simulink model "Dong2015IEEECST1"  (R2016b)
settings: Solver=VariableStepAuto  StartTime=0.0001  StopTime=180  FixedStep=0.01  RelTol=1e-6  AbsTol=1e-6
undefined symbols (not defined in the file or in its folder): A, A_xi, B_h, b_h, B_hv, b_hv, B_xi, dfcn_ht, fcn_ht, fcn_xi, theta0, theta1, xi0
settings Model: Creator=xxx  LastModifiedBy=xxx

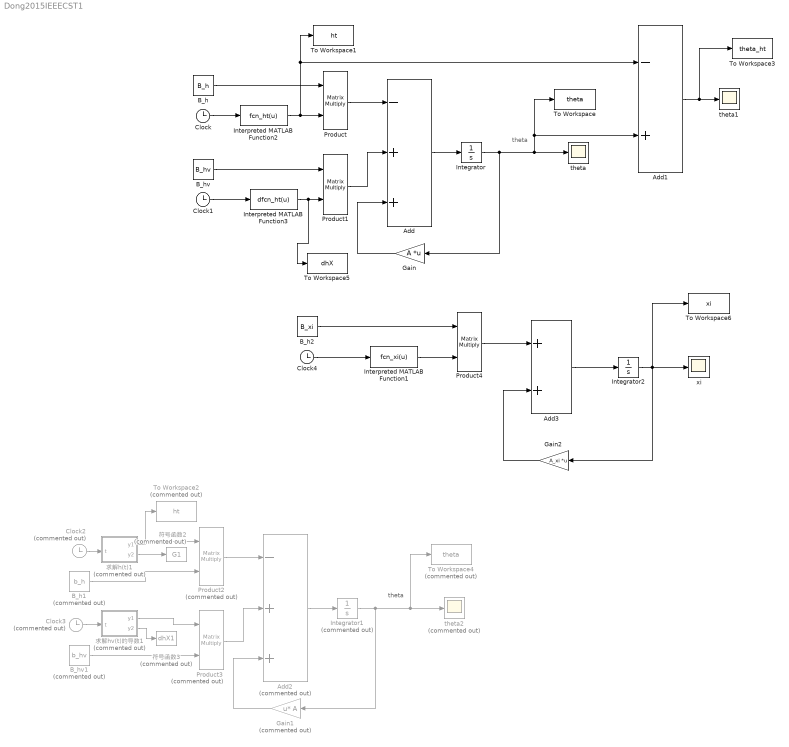
== system Dong2015IEEECST1 ==
  note: theta
  note: theta
  Add : Sum  Inputs=-++
  Add1 : Sum  Inputs=-+
  Add2 : Sum  Commented=on  Inputs=-++
  Add3 : Sum
  B_h : Constant  Value=B_h
  B_h1 : Constant  Commented=on  Value=b_h
  B_h2 : Constant  Value=B_xi
  B_hv : Constant  Value=B_hv
  B_hv1 : Constant  Commented=on  Value=b_hv
  Clock : Clock
  Clock1 : Clock
  Clock2 : Clock  Commented=on
  Clock3 : Clock  Commented=on
  Clock4 : Clock
  Gain : Gain  Gain=A  Multiplication=Matrix(K*u)
  Gain1 : Gain  Commented=on  Gain=A  Multiplication=Matrix(u*K)
  Gain2 : Gain  Gain=A_xi  Multiplication=Matrix(K*u)
  Integrator : Integrator  InitialCondition=theta0
  Integrator1 : Integrator  Commented=on  InitialCondition=theta1
  Integrator2 : Integrator  InitialCondition=xi0
  Interpreted MATLAB Function1 : MATLABFcn  MATLABFcn=fcn_xi(u)
  Interpreted MATLAB Function2 : MATLABFcn  MATLABFcn=fcn_ht(u)
  Interpreted MATLAB Function3 : MATLABFcn  MATLABFcn=dfcn_ht(u)
  Product : Product  Multiplication=Matrix(*)
  Product1 : Product  Multiplication=Matrix(*)
  Product2 : Product  Commented=on  Multiplication=Matrix(*)
  Product3 : Product  Commented=on  Multiplication=Matrix(*)
  Product4 : Product  Multiplication=Matrix(*)
  To Workspace : ToWorkspace  VariableName=theta  SampleTime=-1
      settings: Save2DSignal=2-D array (concatenate along first dimension)
  To Workspace1 : ToWorkspace  VariableName=ht  SampleTime=-1
      settings: Save2DSignal=2-D array (concatenate along first dimension)
  To Workspace2 : ToWorkspace  Commented=on  VariableName=ht  SampleTime=-1
      settings: Save2DSignal=2-D array (concatenate along first dimension)
  To Workspace3 : ToWorkspace  VariableName=theta_ht  SampleTime=-1
      settings: Save2DSignal=2-D array (concatenate along first dimension)
  To Workspace4 : ToWorkspace  Commented=on  VariableName=theta  SampleTime=-1
      settings: Save2DSignal=2-D array (concatenate along first dimension)
  To Workspace5 : ToWorkspace  VariableName=dhX  SampleTime=-1
      settings: Save2DSignal=2-D array (concatenate along first dimension)
  To Workspace6 : ToWorkspace  VariableName=xi  SampleTime=-1
      settings: Save2DSignal=2-D array (concatenate along first dimension)
  theta : Scope
  theta1 : Scope
  theta2 : Scope  Commented=on
  xi : Scope
  求解h(t)1 : MATLAB Function  Commented=on  TreatAsAtomicUnit=on
  求解hv(t)的导数1 : MATLAB Function  Commented=on  TreatAsAtomicUnit=on
  符号函数2 : ToWorkspace  Commented=on  VariableName=G1  SampleTime=-1
      settings: Save2DSignal=2-D array (concatenate along first dimension)
  符号函数3 : ToWorkspace  Commented=on  VariableName=dhX1  SampleTime=-1
      settings: Save2DSignal=2-D array (concatenate along first dimension)
  wires:
  Add/1 -> Integrator/1
  Integrator/1 -> theta/1, Add1/2, To Workspace/1, Gain/1
  Gain/1 -> Add/3
  Clock/1 -> Interpreted MATLAB Function2/1
  求解h(t)1/2(y2) -> 符号函数2/1
  求解h(t)1/1(y1) -> To Workspace2/1, Product2/1
  求解hv(t)的导数1/2(y2) -> 符号函数3/1
  Interpreted MATLAB Function2/1 -> To Workspace1/1, Add1/1, Product/2
  B_h/1 -> Product/1
  Clock1/1 -> Interpreted MATLAB Function3/1
  Interpreted MATLAB Function3/1 -> To Workspace5/1, Product1/2
  B_hv/1 -> Product1/1
  Add1/1 -> To Workspace3/1, theta1/1
  Add2/1 -> Integrator1/1
  Integrator1/1 -> Gain1/1, To Workspace4/1, theta2/1
  Gain1/1 -> Add2/3
  Product2/1 -> Add2/1
  Product3/1 -> Add2/2
  B_h1/1 -> Product2/2
  Clock2/1 -> 求解h(t)1/1(t)
  B_hv1/1 -> Product3/2
  Clock3/1 -> 求解hv(t)的导数1/1(t)
  求解hv(t)的导数1/1(y1) -> Product3/1
  Add3/1 -> Integrator2/1
  Product4/1 -> Add3/1
  Interpreted MATLAB Function1/1 -> Product4/2
  B_h2/1 -> Product4/1
  Clock4/1 -> Interpreted MATLAB Function1/1
  Gain2/1 -> Add3/2
  Integrator2/1 -> To Workspace6/1, xi/1, Gain2/1
  Product/1 -> Add/1
  Product1/1 -> Add/2

== matlab function Dong2015IEEECST1/求解hv(t)的导数1 ==
  data: y1 output; t input; y2 output
function [y1,y2] = fcn_h(t)
r = 7;
omega = 0.214;
g = zeros(1,5);
dh_xX = zeros(1,5);
dh_vX = zeros(1,5);
dh_xY = zeros(1,5);
dh_vY = zeros(1,5);
for i = 1:5
   %% Application1
     g(i) = sign(sin(omega*t/2+pi*(i-1)/5));
    dh_xX(i) = -r*omega*sin((omega*t+2*pi*(i-1)/5)-1)*g(i);%期望编队位置X
    dh_vX(i) = -r*omega^2*cos(omega*t+2*pi*(i-1)/5)*g(i);%期望编队位置Y
    dh_xY(i) = omega*r*cos(omega*t + (2*pi*(i - 1))/5);%期望编队位置Y
    dh_vY(i)= -omega^2*r*sin(omega*t + (2*pi*(i - 1))/5);%期望编队速度Y
    %% Application2
%     dh_xX(i) = r*omega*cos((omega*t+2*pi*(i-1)/5));%期望编队位置X
%     dh_vX(i) = -r*omega^2*sin(omega*t+2*pi*(i-1)/5);%期望编队速度X
%     dh_xY(i) = -r*omega*sin(omega*t+2*pi*(i-1)/5);%期望编队位置Y
%     dh_vY(i)= -r*omega^2*cos(omega*t+2*pi*(i-1)/5);%期望编队速度Y
end
y11 = [dh_vX(:,1) dh_vY(:,1)];
y12 = [dh_vX(:,2) dh_vY(:,2)];
y13 = [dh_vX(:,3) dh_vY(:,3)];
y14 = [dh_vX(:,4) dh_vY(:,4)];
y15 = [dh_vX(:,5) dh_vY(:,5)];

y21 = [dh_xX(:,1) dh_xY(:,1)];
y22 = [dh_xX(:,2) dh_xY(:,2)];
y23 = [dh_xX(:,3) dh_xY(:,3)];
y24 = [dh_xX(:,4) dh_xY(:,4)];
y25 = [dh_xX(:,5) dh_xY(:,5)];
y1 = [y11 y12 y13 y14 y15];
y2 = [y21 y22 y23 y24 y25];

== matlab function Dong2015IEEECST1/求解h(t)1 ==
  data: y1 output; t input; y2 output
function [y1,y2] = fcn_h(t)
r = 7;
omega = 0.214;
g = zeros(1,5);
h_xX = zeros(1,5);
h_vX = zeros(1,5);
h_xY = zeros(1,5);
h_vY = zeros(1,5);
for i = 1:5
         %% Application1
         g(i) = sign(sin(omega*t/2+pi*(i-1)/5));
         h_xX(i) = r*cos((omega*t+2*pi*(i-1)/5)-1)*g(i);%期望编队位置X
         h_vX(i) = -r*omega*sin(omega*t+2*pi*(i-1)/5)*g(i);%期望编队速度X
         h_xY(i) = r*sin(omega*t+2*pi*(i-1)/5);%期望编队位置Y
         h_vY(i)= r*omega*cos(omega*t+2*pi*(i-1)/5);%期望编队速度Y
    
        %% Application2
%         h_xX(i) = r*sin(omega*t+2*pi*(i-1)/5);%期望编队位置X
%         h_vX(i) = r*omega*cos(omega*t+2*pi*(i-1)/5);%期望编队速度X
%         h_xY(i) = r*cos(omega*t+2*pi*(i-1)/5);%期望编队位置Y
%         h_vY(i)= -r*omega*sin(omega*t+2*pi*(i-1)/5);%期望编队速度Y
end
y11 = [h_xX(:,1) h_vX(:,1) h_xY(:,1) h_vY(:,1)];
y12 = [h_xX(:,2) h_vX(:,2) h_xY(:,2) h_vY(:,2)];
y13 = [h_xX(:,3) h_vX(:,3) h_xY(:,3) h_vY(:,3)];
y14 = [h_xX(:,4) h_vX(:,4) h_xY(:,4) h_vY(:,4)];
y15 = [h_xX(:,5) h_vX(:,5) h_xY(:,5) h_vY(:,5)];
y1 = [y11 y12 y13 y14 y15];
y2 = g;
